simulink library "roblocks"  (Simulink 7.7)
settings: Solver=ode45  SolverMode=SingleTasking  StartTime=0.0  StopTime=10.0  RelTol=1e-3
undefined symbols (not defined in the file): angdiff, cam, cond, delta2tr, eul2tr, fkine, jacob0, jacobn, numcols, points, q, qd, qdd, rne, robot, rpy2tr, tr2diff, tr2eul, tr2rpy, transl, trnorm, trotx, z
libraries: simulink3 x2
settings Model: Creator=pic  LastModifiedBy=corkep  ExtModeAutoUpdateStatusClock=off

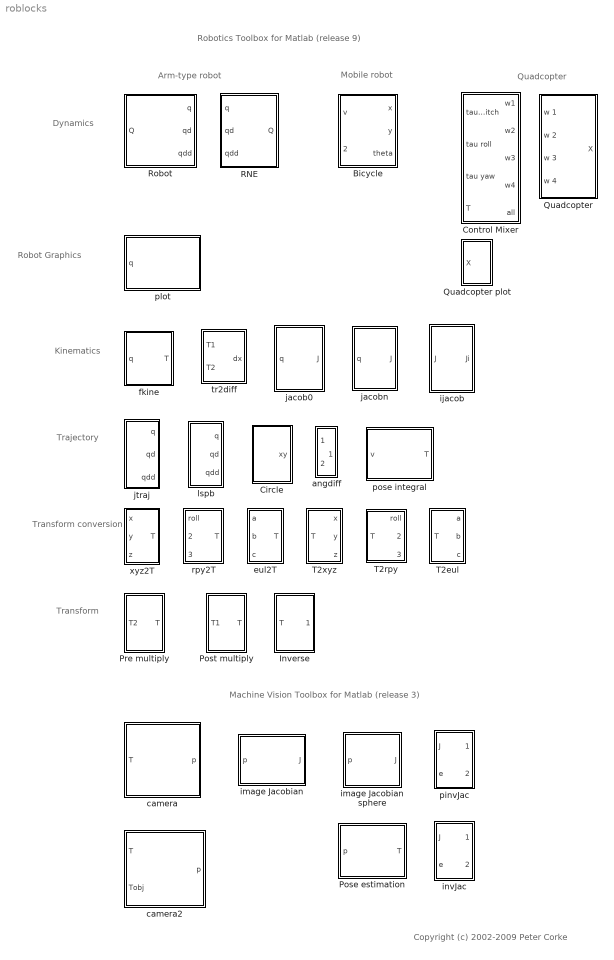
== system roblocks ==
  note: Robotics Toolbox for Matlab (release 9)
  note: Copyright (c) 2002-2009 Peter Corke
  note: Dynamics
  note: Robot
      | Graphics
  note: Kinematics
  note: Transform
      | conversion
  note: Trajectory
  note: Machine Vision Toolbox for Matlab (release 3)
  note: Arm-type robot
  note: Quadcopter
  note: Mobile robot
  note: Transform
  Bicycle : Subsystem  mask{accel=1, vlim=1, alim=2, x0=[0, 0, 0], handbrake=0}
      mask prompts: accel "Acceleration"; vlim "Velocity limit"; alim "Steering limits"; x0 "Initial state (x, y, theta)"
  Circle : Subsystem  mask{radius=1, freq=0.2}
      mask prompts: freq "Frequency (rev/s)"
  Control Mixer : Subsystem
  Inverse : Subsystem
  Pose estimation : Subsystem  mask{cam=0, P=0}
      mask prompts: cam "Camera"; P "Points (3xN)"
  Post multiply : Subsystem  mask{T2=0}
      mask help: Premultiply incoming transform by a constant transformation
  Pre multiply : Subsystem  mask{T=0}
      mask prompts: T "T1"
      mask help: Post multiply incoming transform by constant transform.
  Quadcopter : Subsystem  mask{quad=0}
      mask prompts: quad "Quadcopter params"
  Quadcopter plot : Subsystem
  RNE : Subsystem  mask{robot=robot, grav=[0 0 9.81]}
      mask prompts: robot "Robot object"; grav "Gravity"
      mask help: Rigid-body inverse dynamics.
      mask init:
      | if isa(robot, 'SerialLink')
      |     n = robot.n
      |     rname = robot.name;
      | else
      |     n = 0;
      |     rname = '';
      | end
      mask Help: Given a robot dynamic model and joint angle, rate and acceleration determine the required joint torque.  Useful for computed and inverse torque control schemes.
      mask Display:
      | port_label('output', 1, 'Q')
      | port_label('input', 1, 'q')
      | port_label('input', 2, 'qd')
      | port_label('input', 3, 'qdd')
      | text(0.9, 0.9,  rname, 'horizontalAlignment', 'right')
  Robot : Subsystem  mask{robot=robot, q0=[0 0 0 0 0 0]}
      mask prompts: robot "Robot object"; q0 "Initial state"
      mask help: Rigid-body dynamic model of robot.
      mask init:
      | if isa(robot, 'SerialLink')
      |     rname = robot.name;
      |     fprintf('**robot name is %s\n', rname);
      | else
      |     rname = '';
      |     n = 0
      | end
      mask Help: Simulates the forward (direct) rigid-body dynamics of the robot described by the given robot object.
      mask Display:
      | port_label('input', 1, 'Q')
      | port_label('output', 1, 'q')
      | port_label('output', 2, 'qd')
      | port_label('output', 3, 'qdd')
      | text(0.1, 0.9,  rname, 'horizontalAlignment', 'left')
  T2eul : Subsystem
      mask Description: Convert transform to Euler angles.
  T2rpy : Subsystem
      mask Description: Convert transform to roll/pitch/yaw angles.
  T2xyz : Subsystem
      mask Description: Convert transform to xyz scalars
  angdiff : Subsystem
  camera : Subsystem  mask{cam=, points=}
      mask prompts: cam "Camera"; points "Points (3xN)"
  camera2 : Subsystem
  eul2T : Subsystem
      mask Description: Convert Euler angles to transform.
  fkine : Subsystem  mask{robot=robot}
      mask prompts: robot "Robot object"
      mask help: Robot forward kinematics.
      mask Help: Compute homogeneous transform for robot end-effector given joint angles.
      mask Display:
      | port_label('input', 1, 'q')
      | port_label('output', 1, 'T')
      | text(0.9, 0.9, robot.name,  'horizontalAlignment', 'right')
  ijacob : Subsystem
      mask Description:
      | Robot inverse Jacobian for world coordinates.
      | 
      | Only valid for square jacobians (ie/ 6DOF robots)
      mask Display:
      | text(0.4, 0.7, 'J', 'verticalAlignment', 'top', 'horizontalAlignment', 'left')
      | text(0.65, 0.65, '-1', 'verticalAlignment', 'bottom', 'horizontalAlignment', 'right')
      | port_label('input', 1, 'J');
      | port_label('output', 1, 'Ji')
  image Jacobian : Subsystem  mask{cam=, z=}
      mask prompts: cam "Camera"; z "Assumed depth (m)"
  image Jacobian sphere : Subsystem
  invJac : Subsystem
  "jacob0 " : Subsystem  mask{robot=robot}
      mask prompts: robot "Robot object"
      mask help: Robot Jacobian for end-effector coordinates
      mask init:
      | n=robot.n;
      mask Display:
      | text(0.4, 0.7, 'J', 'verticalAlignment', 'top', 'horizontalAlignment', 'left')
      | text(0.4, 0.7, '0', 'verticalAlignment', 'bottom', 'horizontalAlignment', 'right')
      | text(0.5, 0.2, robot.name,  'horizontalAlignment', 'center')
      | port_label('input', 1, 'q')
      | port_label('output', 1, 'J')
  jacobn : Subsystem  mask{robot=robot}
      mask prompts: robot "Robot object"
      mask help: Robot Jacobian for end-effector coordinates
      mask init:
      | n=robot.n;
      mask Display:
      | text(0.5, 0.4, 'J', 'verticalAlignment', 'top', 'horizontalAlignment', 'left')
      | text(0.5, 0.4, 'n', 'verticalAlignment', 'bottom', 'horizontalAlignment', 'right')
      | text(0.9, 0.9, robot.name,  'horizontalAlignment', 'right')
      | port_label('input', 1, 'q')
      | port_label('output', 1, 'J')
  jtraj : Subsystem  mask{q0=[0 0 0 0 0 0], qf=[pi/4 pi/2 -pi/2 0 0 0], tmax=10}
      mask help: Joint interpolated trajectory.
      mask init:
      | n = length(q0);
      | if length(q0) ~= length(qf) ,
      |  error('q0 and qf must be same length')
      | end
      | t=[0:100]'/100*tmax;
      | [q,qd,qdd] = jtraj(q0, qf, t);
      mask Help:
      | Generate quintic polynomial to move from initial to final joint angles as specified.  Initial and final velocity are assumed to be zero.
      | 
      | Outputs joint angles as well as joint angle rates.
      mask Display:
      | port_label('output', 1, 'q')
      | port_label('output', 2, 'qd')
      | port_label('output', 3, 'qdd')
  lspb : Subsystem  AncestorBlock=roblocks/jtraj  mask{q0=[0 0 0 0 0 0], qf=[pi/4 pi/2 -pi/2 0 0 0], tmax=10}
      mask help: Joint interpolated trajectory.
      mask init:
      | n = length(q0);
      | if length(q0) ~= length(qf) ,
      |  error('q0 and qf must be same length')
      | end
      | t=[0:1000]'/1000*tmax;
      | [q,qd,qdd] = lspb(q0, qf, t);
      mask Help:
      | Generate quintic polynomial to move from initial to final joint angles as specified.  Initial and final velocity are assumed to be zero.
      | 
      | Outputs joint angles as well as joint angle rates.
      mask Display:
      | port_label('output', 1, 'q')
      | port_label('output', 2, 'qd')
      | port_label('output', 3, 'qdd')
  pinvJac : Subsystem
  plot : Subsystem  mask{robot=robot}
      mask prompts: robot "Name of robot"
      mask help: Graphical robot display.
      mask init:
      | if isa(robot, 'SerialLink')
      |     plot(robot,zeros(1,robot.n));
      | rname = robot.name;
      | fprintf('**robot name is %s\n', rname);
      | else
      |     rname = '';
      | end
      mask Help: This block graphically displays the named robot
      mask Display:
      | text(0.5, 0.9,  rname, 'horizontalAlignment', 'center')
      | port_label('input', 1, 'q')
  pose integral : Subsystem  mask{T0=transl(1,1,-3)*trotx(0.2), dt=0.02}
      mask prompts: T0 "Initial pose (hom transform)"; dt "Sample interval (s)"
  rpy2T : Subsystem
      mask Description: Convert roll/pitch/yaw angles to transform.
  tr2diff : Subsystem  mask{robot=robot}
      mask prompts: robot "Robot object"
      mask help: Robot forward kinematics.
      mask Help: Compute homogeneous transform for robot end-effector given joint angles.
      mask Display:
      | port_label('input', 1, 'T1')
      | port_label('input', 2, 'T2')
      | port_label('output', 1, 'dx')
  xyz2T : Subsystem
      mask Description: Convert xyz scalars to transform.

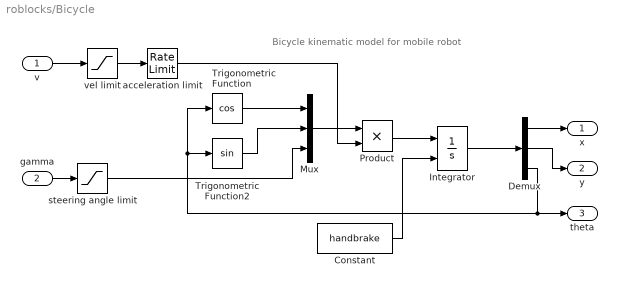
== system roblocks/Bicycle ==
  note: Bicycle kinematic model for mobile robot
  v : Inport
  gamma : Inport  Port=2
  Constant : Constant  Value=handbrake
  Demux : Demux  Outputs=3
  Integrator : Integrator  ExternalReset=level  InitialCondition=x0
  Mux : Mux  Inputs=3
  Product : Product  RndMeth=Zero
  Trigonometric Function : Trigonometry  Operator=cos
  Trigonometric Function2 : Trigonometry
  acceleration limit : RateLimiter  RisingSlewLimit=accel  FallingSlewLimit=-accel  SampleTimeMode=inherited
  steering angle limit : Saturate  UpperLimit=alim  LowerLimit=-alim
  vel limit : Saturate  UpperLimit=vlim  LowerLimit=-vlim
  x : Outport
  y : Outport  Port=2
  theta : Outport  Port=3
  wires:
  Trigonometric Function/1 -> Mux/1
  acceleration limit/1 -> Product/2
  Product/1 -> Integrator/1
  Integrator/1 -> Demux/1
  Demux/3 -> Trigonometric Function/1, Trigonometric Function2/1, theta/1
  Demux/1 -> x/1
  Demux/2 -> y/1
  gamma/1 -> steering angle limit/1
  v/1 -> vel limit/1
  Mux/1 -> Product/1
  vel limit/1 -> acceleration limit/1
  Trigonometric Function2/1 -> Mux/2
  steering angle limit/1 -> Mux/3
  Constant/1 -> Integrator/2

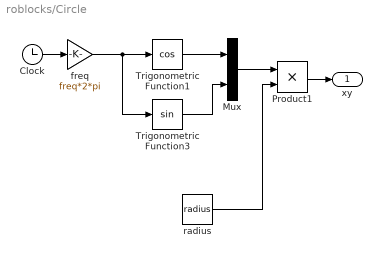
== system roblocks/Circle ==
  Clock : Clock
      settings: Decimation=10
  Mux : Mux  Inputs=2
  Product1 : Product  RndMeth=Zero
  Trigonometric Function1 : Trigonometry  Operator=cos
  Trigonometric Function3 : Trigonometry
  freq : Gain  Gain=freq*2*pi
  radius : Constant  Value=radius
  xy : Outport
  wires:
  freq/1 -> Trigonometric Function3/1, Trigonometric Function1/1
  Product1/1 -> xy/1
  Clock/1 -> freq/1
  radius/1 -> Product1/2
  Mux/1 -> Product1/1
  Trigonometric Function1/1 -> Mux/1
  Trigonometric Function3/1 -> Mux/2

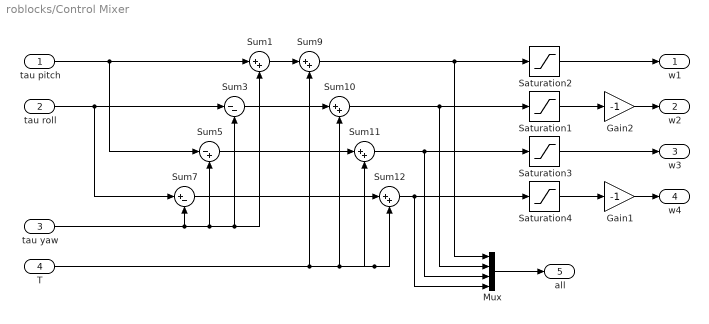
== system roblocks/Control Mixer ==
  tau pitch : Inport
  tau roll : Inport  Port=2
  tau yaw : Inport  Port=3
  T : Inport  Port=4
  Gain1 : Gain  Gain=-1
  Gain2 : Gain  Gain=-1
  Mux : Mux
  Saturation{1..4} (4 alike) : Saturate  UpperLimit=1000  LowerLimit=700
  Sum{1,9..12} (5 alike) : Sum  Inputs=|++  SaturateOnIntegerOverflow=on  InputSameDT=on  OutDataTypeStr=Inherit: Same as first input
  Sum3 : Sum  Inputs=|--  SaturateOnIntegerOverflow=on  InputSameDT=on  OutDataTypeStr=Inherit: Same as first input
  Sum5 : Sum  Inputs=|-+  SaturateOnIntegerOverflow=on  InputSameDT=on  OutDataTypeStr=Inherit: Same as first input
  Sum7 : Sum  Inputs=|+-  SaturateOnIntegerOverflow=on  InputSameDT=on  OutDataTypeStr=Inherit: Same as first input
  w1 : Outport
  w2 : Outport  Port=2
  w3 : Outport  Port=3
  w4 : Outport  Port=4
  all : Outport  Port=5
  wires:
  tau yaw/1 -> Sum7/2, Sum5/2, Sum3/2, Sum1/2
  Saturation2/1 -> w1/1
  Saturation1/1 -> Gain2/1
  Saturation3/1 -> w3/1
  Saturation4/1 -> Gain1/1
  tau pitch/1 -> Sum1/1, Sum5/1
  Sum1/1 -> Sum9/1
  Sum3/1 -> Sum10/1
  Sum5/1 -> Sum11/1
  Sum7/1 -> Sum12/1
  Sum9/1 -> Saturation2/1, Mux/1
  Sum10/1 -> Saturation1/1, Mux/2
  Sum11/1 -> Saturation3/1, Mux/3
  Sum12/1 -> Saturation4/1, Mux/4
  T/1 -> Sum12/2, Sum11/2, Sum10/2, Sum9/2
  tau roll/1 -> Sum3/1, Sum7/1
  Mux/1 -> all/1
  Gain2/1 -> w2/1
  Gain1/1 -> w4/1

== system roblocks/Inverse ==
  T : Inport
  MATLAB Fcn : MATLABFcn  MATLABFcn=inv(u)  OutputDimensions=[4,4]  Output1D=off
  invT : Outport
  wires:
  T/1 -> MATLAB Fcn/1
  MATLAB Fcn/1 -> invT/1

== system roblocks/Pose estimation ==
  p : Inport
  MATLAB Fcn : MATLABFcn  MATLABFcn=cam.estpose(P, u)  OutputDimensions=[4,4]  Output1D=off
  T : Outport
  wires:
  p/1 -> MATLAB Fcn/1
  MATLAB Fcn/1 -> T/1

== system roblocks/Post multiply ==
  T1 : Inport
  Constant : Constant  Value=T2
  Product : Product  Multiplication=Matrix(*)  RndMeth=Zero
  T : Outport
  wires:
  Product/1 -> T/1
  Constant/1 -> Product/2
  T1/1 -> Product/1

== system roblocks/Pre multiply ==
  T2 : Inport
  Constant : Constant  Value=T  VectorParams1D=off
  Product : Product  Multiplication=Matrix(*)  RndMeth=Zero
  T : Outport
  wires:
  Constant/1 -> Product/1
  Product/1 -> T/1
  T2/1 -> Product/2

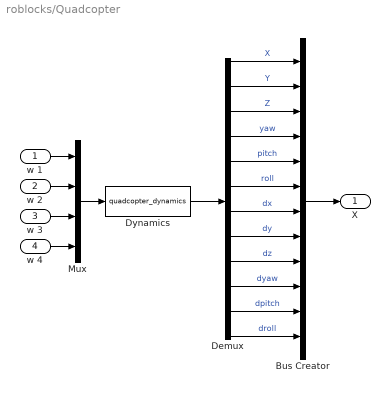
== system roblocks/Quadcopter ==
  w 1 : Inport
  w 2 : Inport  Port=2
  w 3 : Inport  Port=3
  w 4 : Inport  Port=4
  Bus Creator : BusCreator  Inputs='X','Y','Z','yaw','pitch','roll','dx','dy','dz','dyaw','dpitch','droll'
  Demux : Demux  Outputs=12
  Dynamics : S-Function  FunctionName=quadcopter_dynamics  Parameters=quad  EnableBusSupport=off
  Mux : Mux
  X : Outport
  wires:
  Mux/1 -> Dynamics/1
  Demux/1 -> Bus Creator/1  "X"
  Demux/3 -> Bus Creator/3  "Z"
  Demux/4 -> Bus Creator/4  "yaw"
  Demux/5 -> Bus Creator/5  "pitch"
  w 1/1 -> Mux/1
  w 2/1 -> Mux/2
  w 3/1 -> Mux/3
  w 4/1 -> Mux/4
  Demux/7 -> Bus Creator/7  "dx"
  Demux/9 -> Bus Creator/9  "dz"
  Demux/2 -> Bus Creator/2  "Y"
  Demux/6 -> Bus Creator/6  "roll"
  Demux/8 -> Bus Creator/8  "dy"
  Bus Creator/1 -> X/1
  Dynamics/1 -> Demux/1
  Demux/10 -> Bus Creator/10  "dyaw"
  Demux/11 -> Bus Creator/11  "dpitch"
  Demux/12 -> Bus Creator/12  "droll"

== system roblocks/Quadcopter plot ==
  X : Inport
  Bus Selector1 : BusSelector  OutputSignals=X,Y,Z,yaw,pitch,roll  OutputAsBus=on
  Plotter : S-Function  FunctionName=quadcopter_plot  Parameters=[2,10], 1, 1  EnableBusSupport=off
  wires:
  X/1 -> Bus Selector1/1
  Bus Selector1/1 -> Plotter/1

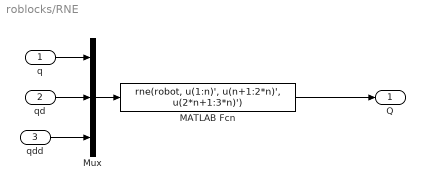
== system roblocks/RNE ==
  q : Inport
  qd : Inport  Port=2
  qdd : Inport  Port=3
  MATLAB Fcn : MATLABFcn  MATLABFcn=rne(robot, u(1:n)', u(n+1:2*n)', u(2*n+1:3*n)')  OutputDimensions=n
  Mux : Mux  Inputs=3
  Q : Outport
  wires:
  MATLAB Fcn/1 -> Q/1
  qdd/1 -> Mux/3
  qd/1 -> Mux/2
  q/1 -> Mux/1
  Mux/1 -> MATLAB Fcn/1

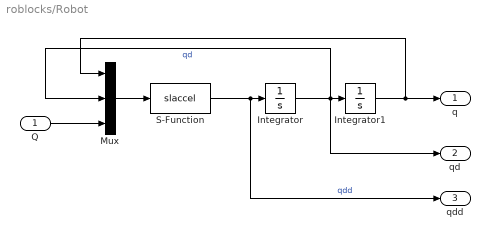
== system roblocks/Robot ==
  Q : Inport
  Integrator : Integrator
  Integrator1 : Integrator
  Mux : Mux  Inputs=3
  S-Function : S-Function  FunctionName=slaccel  Parameters=robot  EnableBusSupport=off
  q : Outport
  qd : Outport  Port=2
  qdd : Outport  Port=3
  wires:
  S-Function/1 -> qdd/1, Integrator/1  "qdd"
  Mux/1 -> S-Function/1
  Integrator/1 -> qd/1, Integrator1/1, Mux/2  "qd"
  Q/1 -> Mux/3
  Integrator1/1 -> q/1, Mux/1

== system roblocks/T2eul ==
  T : Inport
  Demux : Demux  Outputs=3
  MATLAB Fcn : MATLABFcn  MATLABFcn=tr2eul(u)  OutputDimensions=3
  a : Outport
  b : Outport  Port=2
  c : Outport  Port=3
  wires:
  Demux/3 -> c/1
  Demux/2 -> b/1
  Demux/1 -> a/1
  MATLAB Fcn/1 -> Demux/1
  T/1 -> MATLAB Fcn/1

== system roblocks/T2rpy ==
  T : Inport
  Demux : Demux  Outputs=3
  MATLAB Fcn : MATLABFcn  MATLABFcn=tr2rpy(u)  OutputDimensions=3
  roll : Outport
  pitch : Outport  Port=2
  yaw : Outport  Port=3
  wires:
  Demux/3 -> yaw/1
  Demux/2 -> pitch/1
  Demux/1 -> roll/1
  MATLAB Fcn/1 -> Demux/1
  T/1 -> MATLAB Fcn/1

== system roblocks/T2xyz ==
  T : Inport
  Demux : Demux  Outputs=3
  MATLAB Fcn : MATLABFcn  MATLABFcn=transl(u)  OutputDimensions=3
  x : Outport
  y : Outport  Port=2
  z : Outport  Port=3
  wires:
  T/1 -> MATLAB Fcn/1
  MATLAB Fcn/1 -> Demux/1
  Demux/1 -> x/1
  Demux/2 -> y/1
  Demux/3 -> z/1

== system roblocks/angdiff ==
  + : Inport
  - : Inport  Port=2
  MATLAB Fcn : MATLABFcn  MATLABFcn=angdiff(u(1), u(2))
  Mux : Mux  Inputs=2
  d : Outport
  wires:
  +/1 -> Mux/1
  Mux/1 -> MATLAB Fcn/1
  MATLAB Fcn/1 -> d/1
  -/1 -> Mux/2

== system roblocks/camera ==
  T : Inport
  MATLAB Fcn : MATLABFcn  MATLABFcn=cam.plot(points, 'Tcam', u, 'drawnow')  OutputDimensions=[2,numcols(points)]  OutputSignalType=real  Output1D=off
  p : Outport
  wires:
  MATLAB Fcn/1 -> p/1
  T/1 -> MATLAB Fcn/1

== system roblocks/camera2 ==
  T : Inport
  Tobj : Inport  Port=2
  MATLAB Fcn : MATLABFcn  MATLABFcn=cam.plot(points, 'Tcam', u(:,:,1), 'Tobj', u(:,:,2), 'drawnow')  OutputDimensions=[2,numcols(points)]  OutputSignalType=real  Output1D=off
  Matrix Concatenate : Concatenate  Mode=Multidimensional array  ConcatenateDimension=3
  p : Outport
  wires:
  MATLAB Fcn/1 -> p/1
  Matrix Concatenate/1 -> MATLAB Fcn/1
  Tobj/1 -> Matrix Concatenate/2
  T/1 -> Matrix Concatenate/1

== system roblocks/eul2T ==
  a : Inport
  b : Inport  Port=2
  c : Inport  Port=3
  MATLAB Fcn : MATLABFcn  MATLABFcn=eul2tr(u)  OutputDimensions=[4 4]  Output1D=off
  Mux : Mux  Inputs=3
  T : Outport
  wires:
  c/1 -> Mux/3
  MATLAB Fcn/1 -> T/1
  Mux/1 -> MATLAB Fcn/1
  a/1 -> Mux/1
  b/1 -> Mux/2

== system roblocks/fkine ==
  q : Inport
  MATLAB Fcn : MATLABFcn  MATLABFcn=fkine(robot,u)  OutputDimensions=[4 4]  Output1D=off
  T : Outport
  wires:
  q/1 -> MATLAB Fcn/1
  MATLAB Fcn/1 -> T/1

== system roblocks/ijacob ==
  J : Inport
  inverse jacobian : MATLABFcn  MATLABFcn=inv(u)  Output1D=off
  Ji : Outport
  wires:
  inverse jacobian/1 -> Ji/1
  J/1 -> inverse jacobian/1

== system roblocks/image Jacobian ==
  p : Inport
  MATLAB Fcn : MATLABFcn  MATLABFcn=cam.visjac_p(u, z)  Output1D=off
  J : Outport
  wires:
  MATLAB Fcn/1 -> J/1
  p/1 -> MATLAB Fcn/1

== system roblocks/image Jacobian sphere ==
  p : Inport
  MATLAB Fcn : MATLABFcn  MATLABFcn=cam.visjac_p(u, z)  Output1D=off
  J : Outport
  wires:
  MATLAB Fcn/1 -> J/1
  p/1 -> MATLAB Fcn/1

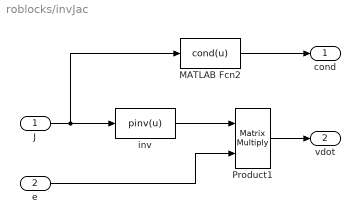
== system roblocks/invJac ==
  J : Inport
  e : Inport  Port=2
  MATLAB Fcn2 : MATLABFcn  MATLABFcn=cond(u)  Output1D=off
  Product1 : Product  Multiplication=Matrix(*)  SaturateOnIntegerOverflow=on  RndMeth=Zero  InputSameDT=on  OutDataTypeStr=Inherit: Same as first input
  inv : MATLABFcn  MATLABFcn=pinv(u)  Output1D=off
  cond : Outport
  vdot : Outport  Port=2
  wires:
  J/1 -> MATLAB Fcn2/1, inv/1
  inv/1 -> Product1/1
  e/1 -> Product1/2
  MATLAB Fcn2/1 -> cond/1
  Product1/1 -> vdot/1

== system roblocks/jacob0  ==
  q : Inport
  MATLAB Fcn : MATLABFcn  MATLABFcn=jacob0(robot,u)  OutputDimensions=[6 n]  Output1D=off
  J : Outport
  wires:
  MATLAB Fcn/1 -> J/1
  q/1 -> MATLAB Fcn/1

== system roblocks/jacobn ==
  q : Inport
  MATLAB Fcn : MATLABFcn  MATLABFcn=jacobn(robot,u)  OutputDimensions=[6 n]  Output1D=off
  J : Outport
  wires:
  MATLAB Fcn/1 -> J/1
  q/1 -> MATLAB Fcn/1

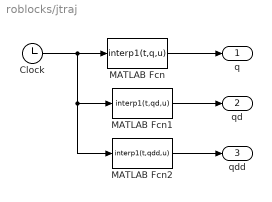
== system roblocks/jtraj ==
  Clock : Clock
      settings: Decimation=10
  MATLAB Fcn : MATLABFcn  MATLABFcn=interp1(t,q,u)  OutputDimensions=n
  MATLAB Fcn1 : MATLABFcn  MATLABFcn=interp1(t,qd,u)  OutputDimensions=n
  MATLAB Fcn2 : MATLABFcn  MATLABFcn=interp1(t,qdd,u)  OutputDimensions=n
  q : Outport
  qd : Outport  Port=2
  qdd : Outport  Port=3
  wires:
  MATLAB Fcn/1 -> q/1
  MATLAB Fcn1/1 -> qd/1
  Clock/1 -> MATLAB Fcn/1, MATLAB Fcn1/1, MATLAB Fcn2/1
  MATLAB Fcn2/1 -> qdd/1

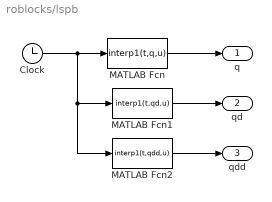
== system roblocks/lspb ==
  Clock : Clock
      settings: Decimation=10
  MATLAB Fcn : MATLABFcn  MATLABFcn=interp1(t,q,u)  OutputDimensions=n
  MATLAB Fcn1 : MATLABFcn  MATLABFcn=interp1(t,qd,u)  OutputDimensions=n
  MATLAB Fcn2 : MATLABFcn  MATLABFcn=interp1(t,qdd,u)  OutputDimensions=n
  q : Outport
  qd : Outport  Port=2
  qdd : Outport  Port=3
  wires:
  MATLAB Fcn2/1 -> qdd/1
  Clock/1 -> MATLAB Fcn2/1, MATLAB Fcn1/1, MATLAB Fcn/1
  MATLAB Fcn1/1 -> qd/1
  MATLAB Fcn/1 -> q/1

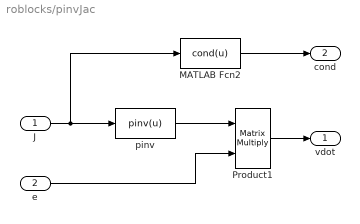
== system roblocks/pinvJac ==
  J : Inport
  e : Inport  Port=2
  MATLAB Fcn2 : MATLABFcn  MATLABFcn=cond(u)  Output1D=off
  Product1 : Product  Multiplication=Matrix(*)  SaturateOnIntegerOverflow=on  RndMeth=Zero  InputSameDT=on  OutDataTypeStr=Inherit: Same as first input
  pinv : MATLABFcn  MATLABFcn=pinv(u)  Output1D=off
  vdot : Outport
  cond : Outport  Port=2
  wires:
  J/1 -> MATLAB Fcn2/1, pinv/1
  pinv/1 -> Product1/1
  e/1 -> Product1/2
  MATLAB Fcn2/1 -> cond/1
  Product1/1 -> vdot/1

== system roblocks/plot ==
  q : Inport
  S-Function : S-Function  FunctionName=slplotbot  Parameters=robot  EnableBusSupport=off
  wires:
  q/1 -> S-Function/1

== system roblocks/pose integral ==
  v : Inport
  MATLAB Fcn3 : MATLABFcn  MATLABFcn=delta2tr(u)  Output1D=off
  Product : Product  Multiplication=Matrix(*)  RndMeth=Zero
  Unit Delay : UnitDelay  X0=T0  SampleTime=dt
  trnorm : MATLABFcn  MATLABFcn=trnorm(u)  Output1D=off
  T : Outport
  wires:
  Product/1 -> trnorm/1
  Unit Delay/1 -> Product/2, T/1
  MATLAB Fcn3/1 -> Product/1
  trnorm/1 -> Unit Delay/1
  v/1 -> MATLAB Fcn3/1

== system roblocks/rpy2T ==
  roll : Inport
  pitch : Inport  Port=2
  yaw : Inport  Port=3
  MATLAB Fcn : MATLABFcn  MATLABFcn=rpy2tr(u)  OutputDimensions=[4 4]  Output1D=off
  Mux : Mux  Inputs=3
  T : Outport
  wires:
  yaw/1 -> Mux/3
  MATLAB Fcn/1 -> T/1
  Mux/1 -> MATLAB Fcn/1
  roll/1 -> Mux/1
  pitch/1 -> Mux/2

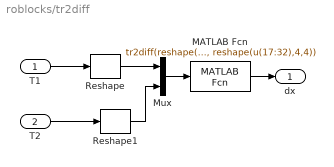
== system roblocks/tr2diff ==
  T1 : Inport
  T2 : Inport  Port=2
  MATLAB Fcn : MATLABFcn  MATLABFcn=tr2diff(reshape(u(1:16),4,4), reshape(u(17:32),4,4))  OutputDimensions=6
  Mux : Mux  Inputs=2
  Reshape : simulink3/Signals & Systems/Reshape  OutputDimensionality=1-D array  OutputDimensions=[1,1]
  Reshape1 : simulink3/Signals & Systems/Reshape  OutputDimensionality=1-D array  OutputDimensions=[1,1]
  dx : Outport
  wires:
  MATLAB Fcn/1 -> dx/1
  T1/1 -> Reshape/1
  T2/1 -> Reshape1/1
  Mux/1 -> MATLAB Fcn/1
  Reshape/1 -> Mux/1
  Reshape1/1 -> Mux/2

== system roblocks/xyz2T ==
  x : Inport
  y : Inport  Port=2
  z : Inport  Port=3
  MATLAB Fcn : MATLABFcn  MATLABFcn=transl(u)  OutputDimensions=[4 4]  Output1D=off
  Mux : Mux  Inputs=3
  T : Outport
  wires:
  y/1 -> Mux/2
  x/1 -> Mux/1
  Mux/1 -> MATLAB Fcn/1
  MATLAB Fcn/1 -> T/1
  z/1 -> Mux/3
